simulink model "new_SAR_ADC"  (R2016a)
settings: Solver=VariableStepAuto  StartTime=0.0  StopTime=inf  RelTol=1e-3
libraries: simulink_extras x11
settings Model: Creator=Lara  LastModifiedBy=Lara

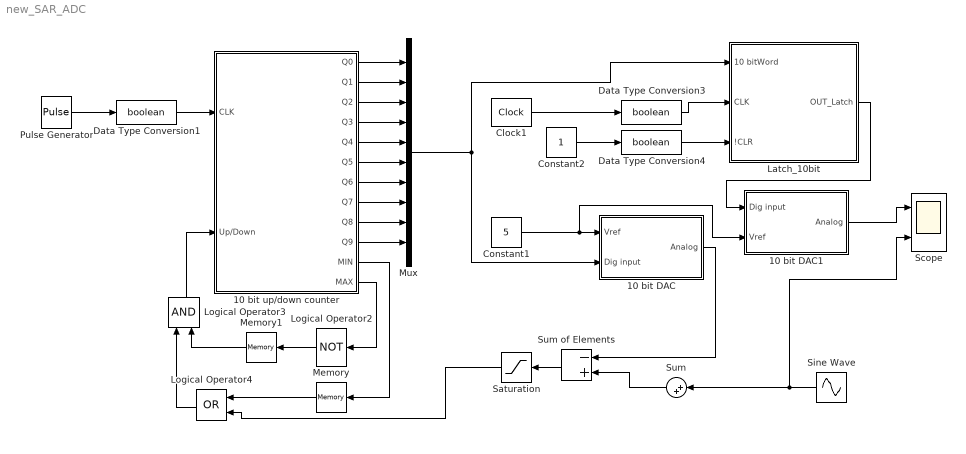
== system new_SAR_ADC ==
  10 bit DAC : Subsystem
  10 bit DAC1 : Subsystem
  10 bit up/down counter : Subsystem
  Clock1 : simulink_extras/Flip Flops/Clock  period=0.0008
  Constant1 : Constant  Value=5
  Constant2 : Constant
  Data Type Conversion1 : DataTypeConversion  OutDataTypeStr=boolean
  Data Type Conversion3 : DataTypeConversion  OutDataTypeStr=boolean
  Data Type Conversion4 : DataTypeConversion  OutDataTypeStr=boolean
  Latch_10bit : Subsystem  AncestorBlock=Digital_8bit_Library/Latch_8bit
  Logical Operator2 : Logic  Operator=NOT  AllPortsSameDT=off  OutDataTypeStr=boolean
  Logical Operator3 : Logic  AllPortsSameDT=off  OutDataTypeStr=boolean
  Logical Operator4 : Logic  Operator=OR  AllPortsSameDT=off  OutDataTypeStr=boolean
  Memory : Memory
  Memory1 : Memory
  Mux : Mux  Inputs=10
  Pulse Generator : DiscretePulseGenerator  PulseType=Time based  Amplitude=5  Period=0.000008  PulseWidth=5
  Saturation : Saturate  UpperLimit=1  LowerLimit=0
  Scope : Scope  NumInputPorts=2
  Sine Wave : Sin  Amplitude=2.49  Bias=2.5  Frequency=10*2*3.142  SampleTime=0
  Sum : Sum  Inputs=|++
  Sum of Elements : Sum  Inputs=-+
  wires:
  Constant1/1 -> 10 bit DAC1/2("Vref "), 10 bit DAC/1("Vref ")
  Mux/1 -> 10 bit DAC/2("Dig input "), Latch_10bit/1(10 bitWord)
  10 bit up/down counter/1(Q0) -> Mux/1
  10 bit up/down counter/2(Q1) -> Mux/2
  10 bit up/down counter/3(Q2) -> Mux/3
  10 bit up/down counter/5(Q4) -> Mux/5
  10 bit up/down counter/4(Q3) -> Mux/4
  10 bit up/down counter/6(Q5) -> Mux/6
  10 bit up/down counter/7(Q6) -> Mux/7
  10 bit up/down counter/8(Q7) -> Mux/8
  10 bit up/down counter/9(Q8) -> Mux/9
  10 bit up/down counter/10(Q9) -> Mux/10
  10 bit up/down counter/12(MAX) -> Logical Operator2/1
  10 bit up/down counter/11(MIN) -> Memory/1
  Logical Operator4/1 -> Logical Operator3/1
  Logical Operator2/1 -> Memory1/1
  Memory1/1 -> Logical Operator3/2
  Memory/1 -> Logical Operator4/1
  Sum of Elements/1 -> Saturation/1
  Saturation/1 -> Logical Operator4/2
  10 bit DAC/1(Analog) -> Sum of Elements/1
  Data Type Conversion1/1 -> 10 bit up/down counter/1(CLK)
  Data Type Conversion3/1 -> Latch_10bit/2(CLK)
  Data Type Conversion4/1 -> Latch_10bit/3(!CLR)
  Constant2/1 -> Data Type Conversion4/1
  Clock1/1 -> Data Type Conversion3/1
  10 bit DAC1/1(Analog) -> Scope/1
  Logical Operator3/1 -> 10 bit up/down counter/2(Up/Down)
  Pulse Generator/1 -> Data Type Conversion1/1
  Sine Wave/1 -> Scope/2, Sum/1
  Sum/1 -> Sum of Elements/2
  Latch_10bit/1(OUT_Latch) -> 10 bit DAC1/1("Dig input ")

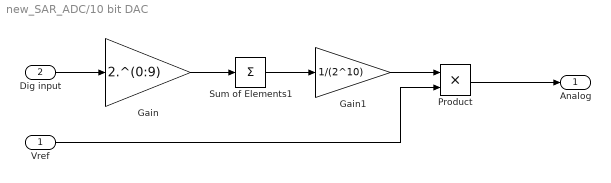
== system new_SAR_ADC/10 bit DAC ==
  "Vref " : Inport
  "Dig input " : Inport  Port=2
  Gain : Gain  Gain=2.^(0:9)
  Gain1 : Gain  Gain=1/(2^10)
  Product : Product  RndMeth=Zero
  Sum of Elements1 : Sum  Inputs=+
  Analog : Outport
  wires:
  "Vref "/1 -> Product/2
  Gain/1 -> Sum of Elements1/1
  Gain1/1 -> Product/1
  "Dig input "/1 -> Gain/1
  Product/1 -> Analog/1
  Sum of Elements1/1 -> Gain1/1

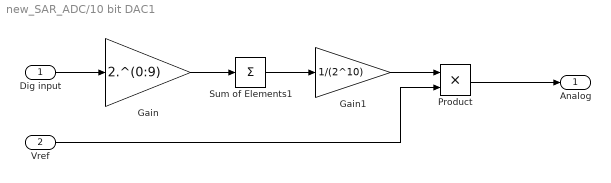
== system new_SAR_ADC/10 bit DAC1 ==
  "Dig input " : Inport
  "Vref " : Inport  Port=2
  Gain : Gain  Gain=2.^(0:9)
  Gain1 : Gain  Gain=1/(2^10)
  Product : Product  RndMeth=Zero
  Sum of Elements1 : Sum  Inputs=+
  Analog : Outport
  wires:
  "Vref "/1 -> Product/2
  Gain/1 -> Sum of Elements1/1
  Gain1/1 -> Product/1
  "Dig input "/1 -> Gain/1
  Product/1 -> Analog/1
  Sum of Elements1/1 -> Gain1/1

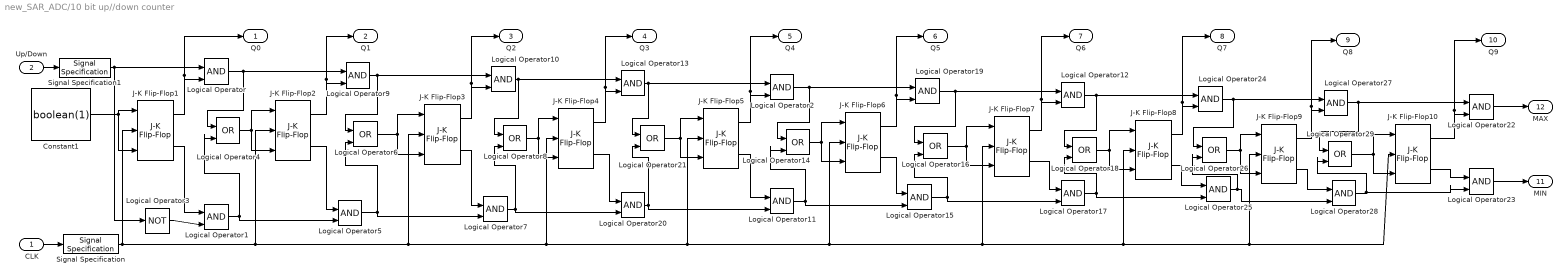
== system new_SAR_ADC/10 bit up//down counter ==
  CLK : Inport
  Up/Down : Inport  Port=2
  Constant1 : Constant  Value=boolean(1)
  J-K Flip-Flop{1..10} (10 alike) : simulink_extras/Flip Flops/J-K Flip-Flop  initial_condition=0
  Logical Operator{,1..2,5,7,9..13,15,17,19..20,22..25,27..28} (20 alike) : Logic  IconShape=distinctive  AllPortsSameDT=off  OutDataTypeStr=boolean
  Logical Operator{4,6,8,14,16,18,21,26,29} (9 alike) : Logic  Operator=OR  IconShape=distinctive  AllPortsSameDT=off  OutDataTypeStr=boolean
  Logical Operator3 : Logic  Operator=NOT  IconShape=distinctive  AllPortsSameDT=off  OutDataTypeStr=boolean
  Signal Specification : SignalSpecification  OutDataTypeStr=boolean
  Signal Specification1 : SignalSpecification  OutDataTypeStr=boolean
  Q0 : Outport  InitialOutput=0
  Q1 : Outport  Port=2  InitialOutput=0
  Q2 : Outport  Port=3  InitialOutput=0
  Q3 : Outport  Port=4  InitialOutput=0
  Q4 : Outport  Port=5  InitialOutput=0
  Q5 : Outport  Port=6  InitialOutput=0
  Q6 : Outport  Port=7  InitialOutput=0
  Q7 : Outport  Port=8  InitialOutput=0
  Q8 : Outport  Port=9  InitialOutput=0
  Q9 : Outport  Port=10  InitialOutput=0
  MIN : Outport  Port=11  InitialOutput=0
  MAX : Outport  Port=12  InitialOutput=0
  wires:
  Logical Operator15/1 -> Logical Operator17/2, Logical Operator16/2
  Logical Operator16/1 -> J-K Flip-Flop7/3, J-K Flip-Flop7/1
  Logical Operator20/1 -> Logical Operator11/2, Logical Operator21/2
  Logical Operator14/1 -> J-K Flip-Flop6/3, J-K Flip-Flop6/1
  J-K Flip-Flop10/2 -> Logical Operator23/1
  Signal Specification1/1 -> Logical Operator/1, Logical Operator3/1
  Logical Operator17/1 -> Logical Operator25/2, Logical Operator18/2
  J-K Flip-Flop7/2 -> Logical Operator17/1
  J-K Flip-Flop7/1 -> Q6/1, Logical Operator12/2
  Logical Operator8/1 -> J-K Flip-Flop4/3, J-K Flip-Flop4/1
  J-K Flip-Flop5/1 -> Q4/1, Logical Operator2/2
  Logical Operator28/1 -> Logical Operator23/2, Logical Operator29/2
  Logical Operator26/1 -> J-K Flip-Flop9/3, J-K Flip-Flop9/1
  J-K Flip-Flop9/2 -> Logical Operator28/1
  Logical Operator12/1 -> Logical Operator18/1, Logical Operator24/1
  Logical Operator7/1 -> Logical Operator20/2, Logical Operator8/2
  Logical Operator10/1 -> Logical Operator13/1, Logical Operator8/1
  Logical Operator9/1 -> Logical Operator10/1, Logical Operator6/1
  Logical Operator29/1 -> J-K Flip-Flop10/3, J-K Flip-Flop10/1
  Constant1/1 -> J-K Flip-Flop1/3, J-K Flip-Flop1/1
  Logical Operator6/1 -> J-K Flip-Flop3/3, J-K Flip-Flop3/1
  J-K Flip-Flop4/1 -> Q3/1, Logical Operator13/2
  J-K Flip-Flop2/1 -> Q1/1, Logical Operator9/2
  J-K Flip-Flop5/2 -> Logical Operator11/1
  Logical Operator24/1 -> Logical Operator26/1, Logical Operator27/1
  Logical Operator18/1 -> J-K Flip-Flop8/3, J-K Flip-Flop8/1
  Logical Operator22/1 -> MAX/1
  J-K Flip-Flop3/2 -> Logical Operator7/1
  J-K Flip-Flop9/1 -> Q8/1, Logical Operator27/2
  Logical Operator2/1 -> Logical Operator19/1, Logical Operator14/1
  J-K Flip-Flop1/1 -> Q0/1, Logical Operator/2
  Logical Operator3/1 -> Logical Operator1/2
  Logical Operator21/1 -> J-K Flip-Flop5/3, J-K Flip-Flop5/1
  J-K Flip-Flop8/2 -> Logical Operator25/1
  Signal Specification/1 -> J-K Flip-Flop3/2, J-K Flip-Flop4/2, J-K Flip-Flop5/2, J-K Flip-Flop6/2, J-K Flip-Flop8/2, J-K Flip-Flop10/2, J-K Flip-Flop9/2, J-K Flip-Flop7/2, J-K Flip-Flop2/2, J-K Flip-Flop1/2
  J-K Flip-Flop10/1 -> Q9/1, Logical Operator22/2
  J-K Flip-Flop2/2 -> Logical Operator5/1
  Logical Operator1/1 -> Logical Operator5/2, Logical Operator4/2
  Logical Operator27/1 -> Logical Operator22/1, Logical Operator29/1
  Logical Operator13/1 -> Logical Operator2/1, Logical Operator21/1
  J-K Flip-Flop4/2 -> Logical Operator20/1
  CLK/1 -> Signal Specification/1
  Logical Operator23/1 -> MIN/1
  Up/Down/1 -> Signal Specification1/1
  J-K Flip-Flop6/1 -> Q5/1, Logical Operator19/2
  J-K Flip-Flop1/2 -> Logical Operator1/1
  Logical Operator11/1 -> Logical Operator15/2, Logical Operator14/2
  Logical Operator25/1 -> Logical Operator28/2, Logical Operator26/2
  Logical Operator19/1 -> Logical Operator12/1, Logical Operator16/1
  J-K Flip-Flop3/1 -> Q2/1, Logical Operator10/2
  J-K Flip-Flop6/2 -> Logical Operator15/1
  Logical Operator4/1 -> J-K Flip-Flop2/1, J-K Flip-Flop2/3
  Logical Operator5/1 -> Logical Operator7/2, Logical Operator6/2
  Logical Operator/1 -> Logical Operator9/1, Logical Operator4/1
  J-K Flip-Flop8/1 -> Logical Operator24/2, Q7/1

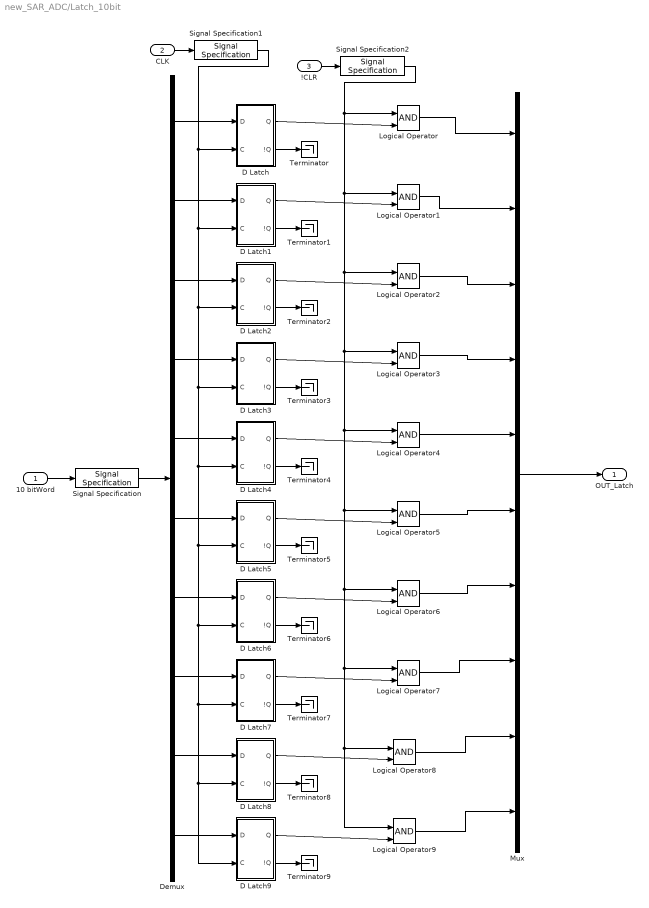
== system new_SAR_ADC/Latch_10bit ==
  10 bitWord : Inport
  CLK : Inport  Port=2
  !CLR : Inport  Port=3
  D Latch : Subsystem  mask(DLatch){}
      mask help: D Latch Flip-Flop Block
      mask Help: web([docroot '/toolbox/simulink/ref_extras/dlatch.html'])
  D Latch1 : Subsystem  mask(DLatch){}
      mask help: D Latch Flip-Flop Block
      mask Help: web([docroot '/toolbox/simulink/ref_extras/dlatch.html'])
  D Latch2 : Subsystem  mask(DLatch){}
      mask help: D Latch Flip-Flop Block
      mask Help: web([docroot '/toolbox/simulink/ref_extras/dlatch.html'])
  D Latch3 : Subsystem  mask(DLatch){}
      mask help: D Latch Flip-Flop Block
      mask Help: web([docroot '/toolbox/simulink/ref_extras/dlatch.html'])
  D Latch4 : Subsystem  mask(DLatch){}
      mask help: D Latch Flip-Flop Block
      mask Help: web([docroot '/toolbox/simulink/ref_extras/dlatch.html'])
  D Latch5 : Subsystem  mask(DLatch){}
      mask help: D Latch Flip-Flop Block
      mask Help: web([docroot '/toolbox/simulink/ref_extras/dlatch.html'])
  D Latch6 : Subsystem  mask(DLatch){}
      mask help: D Latch Flip-Flop Block
      mask Help: web([docroot '/toolbox/simulink/ref_extras/dlatch.html'])
  D Latch7 : Subsystem  mask(DLatch){}
      mask help: D Latch Flip-Flop Block
      mask Help: web([docroot '/toolbox/simulink/ref_extras/dlatch.html'])
  D Latch8 : Subsystem  mask(DLatch){}
      mask help: D Latch Flip-Flop Block
      mask Help: web([docroot '/toolbox/simulink/ref_extras/dlatch.html'])
  D Latch9 : Subsystem  mask(DLatch){}
      mask help: D Latch Flip-Flop Block
      mask Help: web([docroot '/toolbox/simulink/ref_extras/dlatch.html'])
  Demux : Demux  Outputs=10
  Logical Operator{,1..9} (10 alike) : Logic  IconShape=distinctive  AllPortsSameDT=off  OutDataTypeStr=boolean
  Mux : Mux  Inputs=10
  Signal Specification : SignalSpecification  OutDataTypeStr=boolean
  Signal Specification1 : SignalSpecification  OutDataTypeStr=boolean
  Signal Specification2 : SignalSpecification  OutDataTypeStr=boolean
  Terminator{,1..9} (10 alike) : Terminator
  OUT_Latch : Outport
  wires:
  10 bitWord/1 -> Signal Specification/1
  CLK/1 -> Signal Specification1/1
  D Latch/2(!Q) -> Terminator/1
  D Latch1/2(!Q) -> Terminator1/1
  D Latch2/2(!Q) -> Terminator2/1
  D Latch3/2(!Q) -> Terminator3/1
  D Latch4/2(!Q) -> Terminator4/1
  D Latch5/2(!Q) -> Terminator5/1
  D Latch6/2(!Q) -> Terminator6/1
  D Latch7/2(!Q) -> Terminator7/1
  Demux/1 -> D Latch/1(D)
  Demux/2 -> D Latch1/1(D)
  Demux/3 -> D Latch2/1(D)
  Demux/4 -> D Latch3/1(D)
  Demux/5 -> D Latch4/1(D)
  Demux/6 -> D Latch5/1(D)
  Demux/7 -> D Latch6/1(D)
  Demux/8 -> D Latch7/1(D)
  D Latch1/1(Q) -> Logical Operator1/2
  D Latch2/1(Q) -> Logical Operator2/2
  D Latch3/1(Q) -> Logical Operator3/2
  D Latch6/1(Q) -> Logical Operator6/2
  D Latch7/1(Q) -> Logical Operator7/2
  Mux/1 -> OUT_Latch/1
  !CLR/1 -> Signal Specification2/1
  D Latch5/1(Q) -> Logical Operator5/2
  D Latch4/1(Q) -> Logical Operator4/2
  Logical Operator/1 -> Mux/1
  Logical Operator1/1 -> Mux/2
  Logical Operator2/1 -> Mux/3
  Logical Operator3/1 -> Mux/4
  Logical Operator4/1 -> Mux/5
  Logical Operator5/1 -> Mux/6
  Logical Operator6/1 -> Mux/7
  Logical Operator7/1 -> Mux/8
  D Latch/1(Q) -> Logical Operator/2
  Signal Specification/1 -> Demux/1
  Signal Specification1/1 -> D Latch6/2(C), D Latch9/2(C), D Latch8/2(C), D Latch7/2(C), D Latch5/2(C), D Latch4/2(C), D Latch3/2(C), D Latch2/2(C), D Latch1/2(C), D Latch/2(C)
  Signal Specification2/1 -> Logical Operator1/1, Logical Operator2/1, Logical Operator3/1, Logical Operator4/1, Logical Operator9/1, Logical Operator8/1, Logical Operator7/1, Logical Operator6/1, Logical Operator5/1, Logical Operator/1
  Demux/9 -> D Latch8/1(D)
  Demux/10 -> D Latch9/1(D)
  D Latch9/2(!Q) -> Terminator9/1
  D Latch8/2(!Q) -> Terminator8/1
  Logical Operator8/1 -> Mux/9
  Logical Operator9/1 -> Mux/10
  D Latch8/1(Q) -> Logical Operator8/2
  D Latch9/1(Q) -> Logical Operator9/2

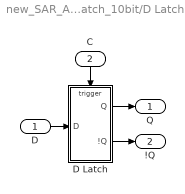
== system new_SAR_ADC/Latch_10bit/D Latch ==
  D : Inport
  C : Inport  Port=2
  D Latch : Subsystem  TreatAsAtomicUnit=on
  Q : Outport  InitialOutput=0
  !Q : Outport  Port=2  InitialOutput=1
  wires:
  C/1 -> D Latch/Trigger
  D Latch/1(Q) -> Q/1
  D/1 -> D Latch/1(D)
  D Latch/2(!Q) -> !Q/1

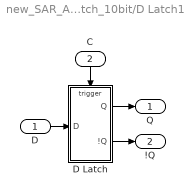
== system new_SAR_ADC/Latch_10bit/D Latch1 ==
  D : Inport
  C : Inport  Port=2
  D Latch : Subsystem  TreatAsAtomicUnit=on
  Q : Outport  InitialOutput=0
  !Q : Outport  Port=2  InitialOutput=1
  wires:
  D Latch/2(!Q) -> !Q/1
  D/1 -> D Latch/1(D)
  D Latch/1(Q) -> Q/1
  C/1 -> D Latch/Trigger

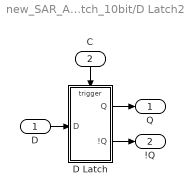
== system new_SAR_ADC/Latch_10bit/D Latch2 ==
  D : Inport
  C : Inport  Port=2
  D Latch : Subsystem  TreatAsAtomicUnit=on
  Q : Outport  InitialOutput=0
  !Q : Outport  Port=2  InitialOutput=1
  wires:
  C/1 -> D Latch/Trigger
  D Latch/1(Q) -> Q/1
  D/1 -> D Latch/1(D)
  D Latch/2(!Q) -> !Q/1

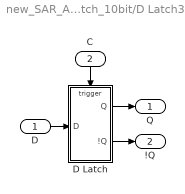
== system new_SAR_ADC/Latch_10bit/D Latch3 ==
  D : Inport
  C : Inport  Port=2
  D Latch : Subsystem  TreatAsAtomicUnit=on
  Q : Outport  InitialOutput=0
  !Q : Outport  Port=2  InitialOutput=1
  wires:
  D Latch/2(!Q) -> !Q/1
  D/1 -> D Latch/1(D)
  D Latch/1(Q) -> Q/1
  C/1 -> D Latch/Trigger

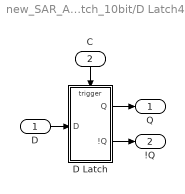
== system new_SAR_ADC/Latch_10bit/D Latch4 ==
  D : Inport
  C : Inport  Port=2
  D Latch : Subsystem  TreatAsAtomicUnit=on
  Q : Outport  InitialOutput=0
  !Q : Outport  Port=2  InitialOutput=1
  wires:
  C/1 -> D Latch/Trigger
  D Latch/1(Q) -> Q/1
  D/1 -> D Latch/1(D)
  D Latch/2(!Q) -> !Q/1

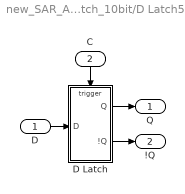
== system new_SAR_ADC/Latch_10bit/D Latch5 ==
  D : Inport
  C : Inport  Port=2
  D Latch : Subsystem  TreatAsAtomicUnit=on
  Q : Outport  InitialOutput=0
  !Q : Outport  Port=2  InitialOutput=1
  wires:
  D Latch/2(!Q) -> !Q/1
  D/1 -> D Latch/1(D)
  D Latch/1(Q) -> Q/1
  C/1 -> D Latch/Trigger

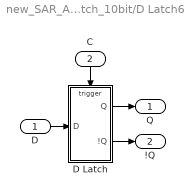
== system new_SAR_ADC/Latch_10bit/D Latch6 ==
  D : Inport
  C : Inport  Port=2
  D Latch : Subsystem  TreatAsAtomicUnit=on
  Q : Outport  InitialOutput=0
  !Q : Outport  Port=2  InitialOutput=1
  wires:
  C/1 -> D Latch/Trigger
  D Latch/1(Q) -> Q/1
  D/1 -> D Latch/1(D)
  D Latch/2(!Q) -> !Q/1

== system new_SAR_ADC/Latch_10bit/D Latch7 ==
  D : Inport
  C : Inport  Port=2
  D Latch : Subsystem  TreatAsAtomicUnit=on
  Q : Outport  InitialOutput=0
  !Q : Outport  Port=2  InitialOutput=1
  wires:
  D Latch/2(!Q) -> !Q/1
  D/1 -> D Latch/1(D)
  D Latch/1(Q) -> Q/1
  C/1 -> D Latch/Trigger

== system new_SAR_ADC/Latch_10bit/D Latch8 ==
  D : Inport
  C : Inport  Port=2
  D Latch : Subsystem  TreatAsAtomicUnit=on
  Q : Outport  InitialOutput=0
  !Q : Outport  Port=2  InitialOutput=1
  wires:
  D Latch/2(!Q) -> !Q/1
  D/1 -> D Latch/1(D)
  D Latch/1(Q) -> Q/1
  C/1 -> D Latch/Trigger

== system new_SAR_ADC/Latch_10bit/D Latch9 ==
  D : Inport
  C : Inport  Port=2
  D Latch : Subsystem  TreatAsAtomicUnit=on
  Q : Outport  InitialOutput=0
  !Q : Outport  Port=2  InitialOutput=1
  wires:
  D Latch/2(!Q) -> !Q/1
  D/1 -> D Latch/1(D)
  D Latch/1(Q) -> Q/1
  C/1 -> D Latch/Trigger

== system new_SAR_ADC/Latch_10bit/D Latch/D Latch ==
  D : Inport
  Trigger : TriggerPort  VariantControl=Variant
  Logic : Logic  Operator=NOT  Inputs=1
  Q : Outport  InitialOutput=0
  !Q : Outport  Port=2  InitialOutput=1
  wires:
  Logic/1 -> !Q/1
  D/1 -> Q/1, Logic/1

== system new_SAR_ADC/Latch_10bit/D Latch1/D Latch ==
  D : Inport
  Trigger : TriggerPort  VariantControl=Variant
  Logic : Logic  Operator=NOT  Inputs=1
  Q : Outport  InitialOutput=0
  !Q : Outport  Port=2  InitialOutput=1
  wires:
  D/1 -> Logic/1, Q/1
  Logic/1 -> !Q/1

== system new_SAR_ADC/Latch_10bit/D Latch2/D Latch ==
  D : Inport
  Trigger : TriggerPort  VariantControl=Variant
  Logic : Logic  Operator=NOT  Inputs=1
  Q : Outport  InitialOutput=0
  !Q : Outport  Port=2  InitialOutput=1
  wires:
  Logic/1 -> !Q/1
  D/1 -> Q/1, Logic/1

== system new_SAR_ADC/Latch_10bit/D Latch3/D Latch ==
  D : Inport
  Trigger : TriggerPort  VariantControl=Variant
  Logic : Logic  Operator=NOT  Inputs=1
  Q : Outport  InitialOutput=0
  !Q : Outport  Port=2  InitialOutput=1
  wires:
  D/1 -> Logic/1, Q/1
  Logic/1 -> !Q/1

== system new_SAR_ADC/Latch_10bit/D Latch4/D Latch ==
  D : Inport
  Trigger : TriggerPort  VariantControl=Variant
  Logic : Logic  Operator=NOT  Inputs=1
  Q : Outport  InitialOutput=0
  !Q : Outport  Port=2  InitialOutput=1
  wires:
  Logic/1 -> !Q/1
  D/1 -> Q/1, Logic/1

== system new_SAR_ADC/Latch_10bit/D Latch5/D Latch ==
  D : Inport
  Trigger : TriggerPort  VariantControl=Variant
  Logic : Logic  Operator=NOT  Inputs=1
  Q : Outport  InitialOutput=0
  !Q : Outport  Port=2  InitialOutput=1
  wires:
  D/1 -> Logic/1, Q/1
  Logic/1 -> !Q/1

== system new_SAR_ADC/Latch_10bit/D Latch6/D Latch ==
  D : Inport
  Trigger : TriggerPort  VariantControl=Variant
  Logic : Logic  Operator=NOT  Inputs=1
  Q : Outport  InitialOutput=0
  !Q : Outport  Port=2  InitialOutput=1
  wires:
  Logic/1 -> !Q/1
  D/1 -> Q/1, Logic/1

== system new_SAR_ADC/Latch_10bit/D Latch7/D Latch ==
  D : Inport
  Trigger : TriggerPort  VariantControl=Variant
  Logic : Logic  Operator=NOT  Inputs=1
  Q : Outport  InitialOutput=0
  !Q : Outport  Port=2  InitialOutput=1
  wires:
  D/1 -> Logic/1, Q/1
  Logic/1 -> !Q/1

== system new_SAR_ADC/Latch_10bit/D Latch8/D Latch ==
  D : Inport
  Trigger : TriggerPort  VariantControl=Variant
  Logic : Logic  Operator=NOT  Inputs=1
  Q : Outport  InitialOutput=0
  !Q : Outport  Port=2  InitialOutput=1
  wires:
  D/1 -> Logic/1, Q/1
  Logic/1 -> !Q/1

== system new_SAR_ADC/Latch_10bit/D Latch9/D Latch ==
  D : Inport
  Trigger : TriggerPort  VariantControl=Variant
  Logic : Logic  Operator=NOT  Inputs=1
  Q : Outport  InitialOutput=0
  !Q : Outport  Port=2  InitialOutput=1
  wires:
  D/1 -> Logic/1, Q/1
  Logic/1 -> !Q/1
